simulink model "pmsm_sim"  (R2018a)
settings: Solver=ode15s  StartTime=0.0  StopTime=1  FixedStep=FastTsample / 10.  RelTol=1e-3
undefined symbols (not defined in the file): EncCntsToRads, MtrCtrlCal_T, MtrCtrlMd_T, MtrParams
libraries: powerlib x16, nesl_utility x12, fl_lib x10, pe_lib x5, pePwmGeneratorTwoLevel x1, powerlib_meascontrol x1
settings Model: Creator=elrobotista  LastModifiedBy=elrobotista
settings OptimizationCC: UseDivisionForNetSlopeComputation=on
settings ModelReferenceCC: EnableRefExpFcnMdlSchedulingChecks=off

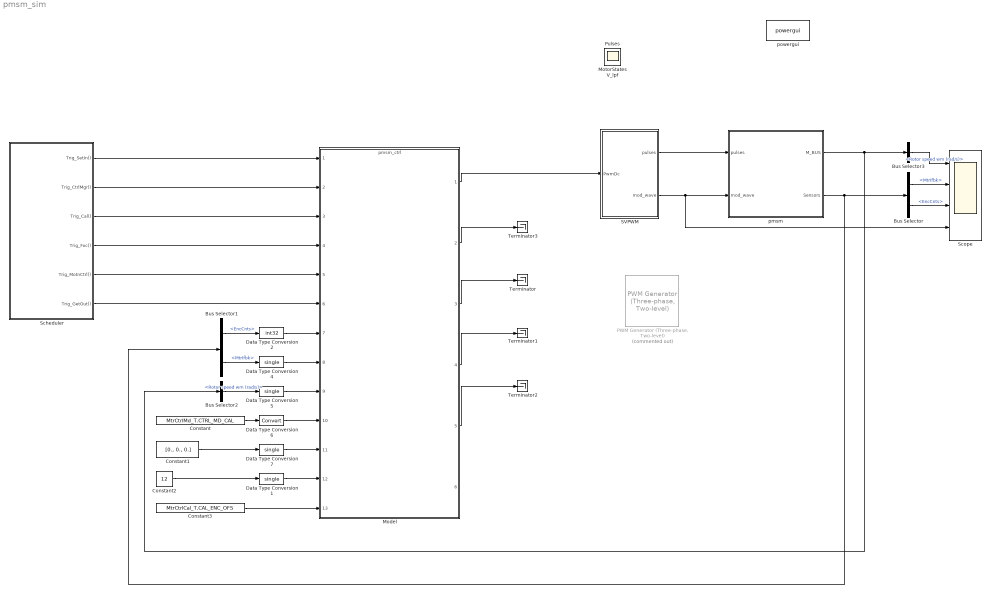
== system pmsm_sim ==
  " Scheduler" : Stateflow chart  TreatAsAtomicUnit=on  SystemSampleTime=1/30e3
  Bus Selector : BusSelector  OutputSignals=MtrIfbk,EncCnts
  Bus Selector1 : BusSelector  OutputSignals=EncCnts,MtrIfbk
  Bus Selector2 : BusSelector  OutputSignals=Rotor speed wm (rad/s)
  Bus Selector3 : BusSelector  OutputSignals=Rotor speed wm (rad/s)
  Constant : Constant  Value=MtrCtrlMd_T.CTRL_MD_CAL
  Constant1 : Constant  Value=[0., 0., 0.]
  Constant2 : Constant  Value=12
  Constant3 : Constant  Value=MtrCtrlCal_T.CAL_ENC_OFS
  Data Type Conversion{1,4..5,7} (4 alike) : DataTypeConversion  OutDataTypeStr=single
  Data Type Conversion2 : DataTypeConversion  OutDataTypeStr=int32
  Data Type Conversion6 : DataTypeConversion
  Model : ModelReference  ModelNameDialog=pmsm_ctrl  SimulationMode=Normal  ShowModelPeriodicEventPorts=on  ModelReferenceVersion=1.728
  "PWM Generator (Three-phase, Two-level)" : pePwmGeneratorTwoLevel/PWM Generator (Three-phase, Two-level)  Commented=on  OverrideUsingVariant=NaturalMode  PWMMode=Continuous PWM (CPWM)  CPWMMode=SPWM: sinusoidal PWM  DPWMMode=60 DPWM: 60 degree discontinuous PWM  fsw=30e3  Ts=5e-5
      settings: SamplingMode=Natural
  SVPWM : Subsystem
  Scope : Scope  NumInputPorts=4
  Terminator{,1..3} (4 alike) : Terminator
  pmsm : Subsystem  Variant=on  VariantControl=Variant1  OverrideUsingVariant=Variant1
  powergui : powerlib/powergui  Priority=1  SimulationMode=Continuous  SampleTime=50e-6  frequency=60  Iterations=50  frequencyindice=0  Pbase=100e6  ErrMax=1e-4  UnitsV=kV  UnitsW=MW  buscounter=0  FunctionMessages=off  echomessages=off  EnableUseOfTLC=off  CurrentSourceSwitches=off  DisableSnubberDevices=off  DisableRonSwitches=off  DisableVfSwitches=off  DisplayEquations=off  SolverType=Tustin/Backward Euler (TBE)  Interpol=off  ExternalGateDelay=off  methode=off  Ts=100  x0status=blocks  SPID=on  SwTol=0  HookPort=off  RestoreLinks=warning  ResistiveCurrentMeasurement=off  Frange=[0:2:500]  Ylog=off  Xlog=on  ShowGrid=off  save=off  variable=ZData  structure=0  ZoomFFT=off  StartTime=0.0  cycles=1  DisplayStyle=1  fundamental=60  FreqAxis=off  MaxFrequency=1000  frequencyindicesteady=1  RmsSteady=1  display=off
  MotorStates : Scope
  Pulses : Scope
  V_lpf : Scope
  wires:
  Bus Selector1/1 -> Data Type Conversion2/1  "<EncCnts>"
  Bus Selector1/2 -> Data Type Conversion4/1  "<MtrIfbk>"
  Constant/1 -> Data Type Conversion6/1
  Bus Selector2/1 -> Data Type Conversion5/1  "<Rotor speed wm (rad/s)>"
  Model/3 -> Terminator/1
  Model/4 -> Terminator1/1
  SVPWM/2(mod_wave) -> Scope/4, pmsm/2("mod_wave ")
  pmsm/1(" M_BUS") -> Bus Selector2/1, Bus Selector3/1
  pmsm/2(" Sensors") -> Bus Selector1/1, Bus Selector/1
  Constant1/1 -> Data Type Conversion7/1
  Model/5 -> Terminator2/1
  " Scheduler"/1(Trig_SetIn()) -> Model/1
  " Scheduler"/2(Trig_CtrlMgr()) -> Model/2
  " Scheduler"/3(Trig_Cal()) -> Model/3
  " Scheduler"/4(Trig_Foc()) -> Model/4
  " Scheduler"/5(Trig_MotnCtrl()) -> Model/5
  " Scheduler"/6(Trig_GetOut()) -> Model/6
  Data Type Conversion2/1 -> Model/7
  Data Type Conversion4/1 -> Model/8
  Data Type Conversion5/1 -> Model/9
  Data Type Conversion6/1 -> Model/10
  Data Type Conversion7/1 -> Model/11
  Data Type Conversion1/1 -> Model/12
  Model/1 -> SVPWM/1(PwmDc)
  Bus Selector/2 -> Scope/3  "<EncCnts>"
  Bus Selector/1 -> Scope/2  "<MtrIfbk>"
  Bus Selector3/1 -> Scope/1  "<Rotor speed wm (rad/s)>"
  Model/2 -> Terminator3/1
  SVPWM/1(pulses) -> pmsm/1("pulses ")
  Constant2/1 -> Data Type Conversion1/1
  Constant3/1 -> Model/13

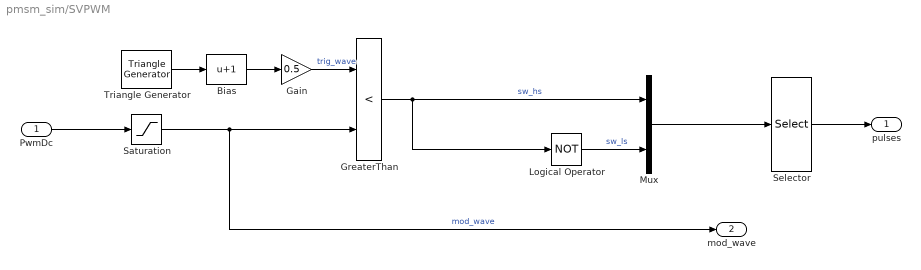
== system pmsm_sim/SVPWM ==
  PwmDc : Inport
  Bias : Bias  Bias=1
  Gain : Gain  Gain=0.5
  GreaterThan : RelationalOperator  Operator=<  OutDataTypeStr=boolean  RndMeth=Simplest
  Logical Operator : Logic  Operator=NOT  AllPortsSameDT=off  OutDataTypeStr=boolean
  Mux : Mux  Inputs=2
  Saturation : Saturate  UpperLimit=1  LowerLimit=0
  Selector : Selector  InputPortWidth=6  IndexOptions=Index vector (dialog)  Indices=[1 4 2 5 3 6]  OutputSizes=1
  Triangle Generator : powerlib_meascontrol/Pulse & Signal Generators/Triangle Generator  Freq=20e3  Phase=90  Ts=0
      settings: SourceProductName=Simscape Electrical
  pulses : Outport  VectorParamsAs1DForOutWhenUnconnected=on
  mod_wave : Outport  Port=2  VectorParamsAs1DForOutWhenUnconnected=on
  wires:
  Triangle Generator/1 -> Bias/1
  Bias/1 -> Gain/1
  Gain/1 -> GreaterThan/1  "trig_wave"
  Saturation/1 -> GreaterThan/2, mod_wave/1  "mod_wave"
  Logical Operator/1 -> Mux/2  "sw_ls"
  GreaterThan/1 -> Logical Operator/1, Mux/1  "sw_hs"
  PwmDc/1 -> Saturation/1
  Selector/1 -> pulses/1
  Mux/1 -> Selector/1

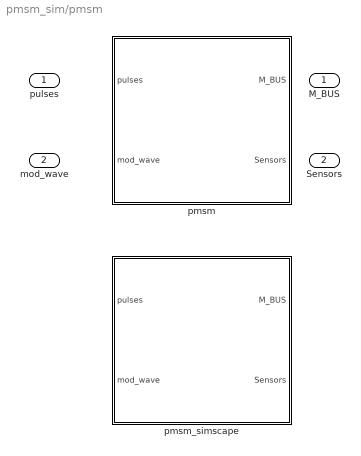
== system pmsm_sim/pmsm ==
  "pulses " : Inport
  "mod_wave " : Inport  Port=2
  pmsm : Subsystem  VariantControl=Variant2
  pmsm_simscape : Subsystem  VariantControl=Variant1
  " M_BUS" : Outport
  " Sensors" : Outport  Port=2

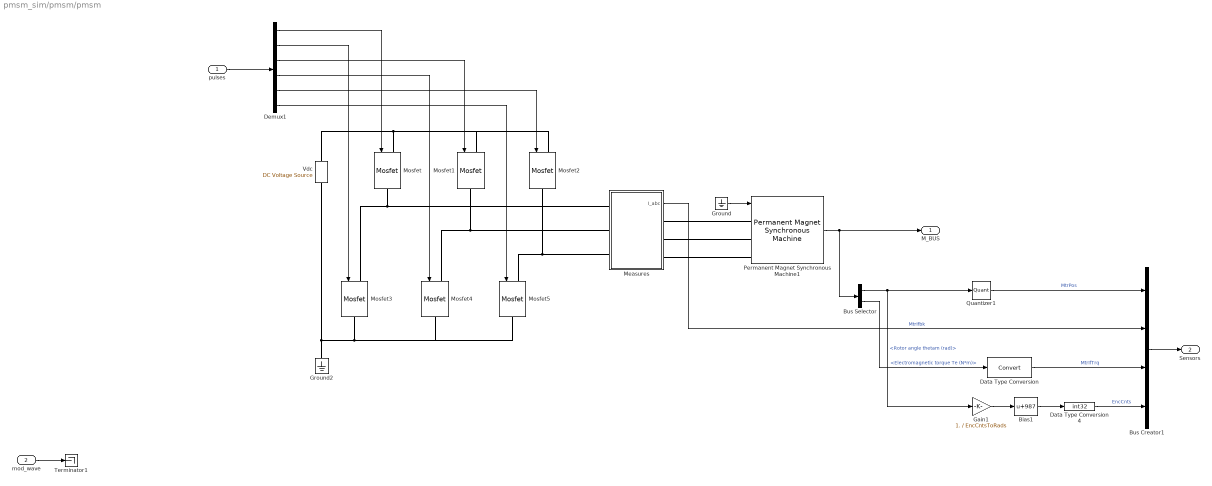
== system pmsm_sim/pmsm/pmsm ==
  pulses : Inport
  mod_wave : Inport  Port=2
  Bias1 : Bias  Bias=987
  Bus Creator1 : BusCreator  Inputs=4
  Bus Selector : BusSelector  OutputSignals=Rotor angle thetam (rad),Electromagnetic torque Te (N*m)
  Data Type Conversion : DataTypeConversion
  Data Type Conversion4 : DataTypeConversion  OutDataTypeStr=int32
  Demux1 : Demux  Outputs=6
  Gain1 : Gain  Gain=1. / EncCntsToRads  OutDataTypeStr=Inherit: Inherit via back propagation
      settings: AttributesFormatString=%<Gain>
  Ground : Ground
  Ground2 : powerlib/Elements/Ground  LConnTagsString=a
      settings: SourceProductName=Simscape Electrical
  Measures : Subsystem
  Mosfet{,1..5} (6 alike) : powerlib/Power Electronics/Mosfet  Ron=0.1  Lon=0  Rd=0.01  Vfd=0  IC=0  Rs=1e5  Cs=inf  Measurements=off
  Permanent Magnet Synchronous Machine1 : powerlib/Machines/Permanent Magnet Synchronous Machine  NbPhases=3  FluxDistribution=Sinusoidal  RotorType=Salient-pole  MechanicalLoad=Torque Tm  PresetModel=No  ShowDetailedParameters=on  MeasurementBus=off  Resistance=MtrParams.Rs  Inductance=8.5e-3  dqInductances=[MtrParams.Ld, MtrParams.Lq]  La=MtrParams.Ls  MachineConstant=Torque Constant (N.m / A_peak)  Flux=0.0058333  VoltageCst=4.2322  TorqueCst=MtrParams.Ktrq  Flat=120  Mechanical=[MtrParams.Jm, MtrParams.Kf, MtrParams.Poles, 0]  PolePairs=4  InitialConditions=[0,0, 0,0]  InitialConditions5ph=[0 0 0 0 0 0]  TsPowergui=0  TsBlock=-1  RefAngle=90 degrees behind phase A axis (modified Park)
  Quantizer1 : Quantizer  QuantizationInterval=2 * pi / MtrParams.EncCnts
  Terminator1 : Terminator
  Vdc : powerlib/Electrical Sources/DC Voltage Source  Amplitude=MtrParams.Vdc  Measurements=None
      settings: SourceProductName=Simscape Electrical
  M_BUS : Outport
  Sensors : Outport  Port=2
  wires:
  Ground/1 -> Permanent Magnet Synchronous Machine1/1
  Permanent Magnet Synchronous Machine1/1 -> Bus Selector/1, M_BUS/1
  Bus Selector/1 -> Quantizer1/1, Gain1/1  "<Rotor angle thetam (rad)>"
  Measures/1(I_abc) -> Bus Creator1/2  "MtrIfbk"
  pulses/1 -> Demux1/1
  Quantizer1/1 -> Bus Creator1/1  "MtrPos"
  Bias1/1 -> Data Type Conversion4/1
  Gain1/1 -> Bias1/1
  Bus Selector/2 -> Data Type Conversion/1  "<Electromagnetic torque Te (N*m)>"
  Bus Creator1/1 -> Sensors/1
  Data Type Conversion4/1 -> Bus Creator1/4  "EncCnts"
  Data Type Conversion/1 -> Bus Creator1/3  "MtrIfTrq"
  mod_wave/1 -> Terminator1/1
  Demux1/1 -> Mosfet/1
  Demux1/2 -> Mosfet3/1
  Demux1/3 -> Mosfet1/1
  Demux1/4 -> Mosfet4/1
  Demux1/5 -> Mosfet2/1
  Demux1/6 -> Mosfet5/1
  connections:
  Permanent Magnet Synchronous Machine1/LConn3 -- Measures/RConn3
  Permanent Magnet Synchronous Machine1/LConn2 -- Measures/RConn2
  Permanent Magnet Synchronous Machine1/LConn1 -- Measures/RConn1
  Mosfet5/RConn1 -- Mosfet4/RConn1 -- Mosfet3/RConn1 -- Vdc/LConn1 -- Ground2/LConn1
  Mosfet5/LConn1 -- Measures/LConn3 -- Mosfet2/RConn1
  Mosfet2/LConn1 -- Mosfet1/LConn1 -- Mosfet/LConn1 -- Vdc/RConn1
  Mosfet4/LConn1 -- Measures/LConn2 -- Mosfet1/RConn1
  Mosfet3/LConn1 -- Measures/LConn1 -- Mosfet/RConn1

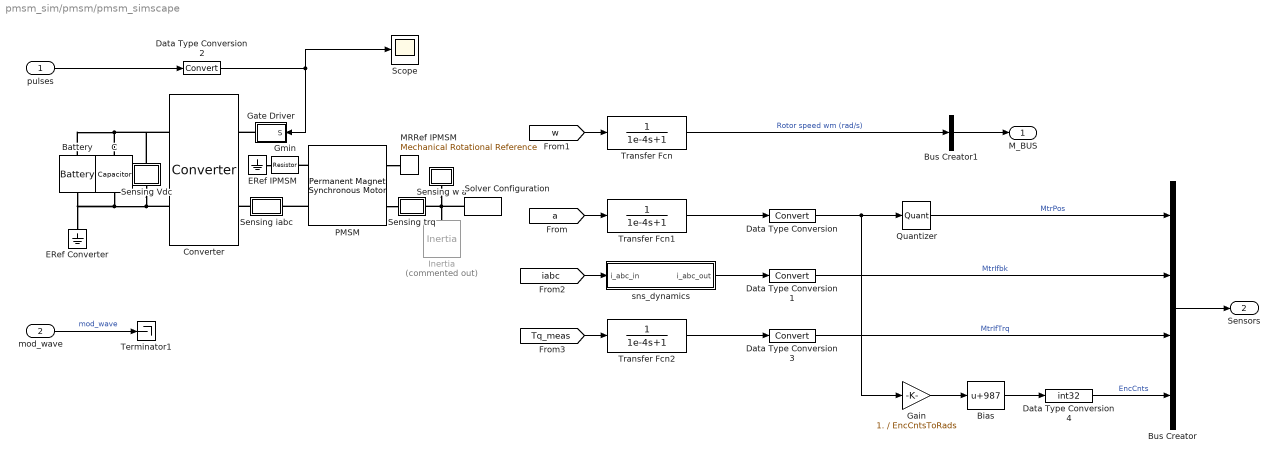
== system pmsm_sim/pmsm/pmsm_simscape ==
  pulses : Inport
  mod_wave : Inport  Port=2
  Battery : pe_lib/Sources/Battery  Vnom=MtrParams.Vdc V  R1=0.001 Ohm  prm_AH=1  AH=200 hr*A  V1=290 V  AH1=50 hr*A  prm_R2=1  R2=2000 Ohm  prm_dyn=1  Rp1=0.005 Ohm  tau1=30 s  Rp2=0.005 Ohm  tau2=30 s  prm_fade=1  N_fade=100  AH_fade=45 hr*A  R1_fade=2.02 Ohm  V1_fade=10.35 V  i_specify=off  i_priority=None  i=0 A  i_nominal_specify=off  i_nominal_unit=A  i_nominal_value=1  v_specify=off  v_priority=None  v=0 V  v_nominal_specify=off  v_nominal_unit=V  v_nominal_value=1  charge_specify=on  charge_priority=High  charge=200 hr*A  charge_nominal_specify=off  charge_nominal_unit=hr*A  charge_nominal_value=1  num_cycles_specify=off  num_cycles_priority=High  num_cycles=0  num_cycles_nominal_specify=off  num_cycles_nominal_unit=1  num_cycles_nominal_value=1  thermal_mass=30000 J/K  Tmeas=298.15 K  Vnom_T2=12 V  R1_T2=2.2 Ohm  V1_T2=11.4 V  R2_T2=2200 Ohm  Rp1_T2=0.005 Ohm  tau1_T2=30 s  Rp2_T2=0.005 Ohm  tau2_T2=30 s  Tmeas2=273.15 K  temperature_specify=off  temperature_priority=High  temperature=298.15 K  temperature_nominal_specify=off  temperature_nominal_unit=K  temperature_nominal_value=1
      settings: SourceProductName=Simscape Power Systems  SourceProductBaseCode=PS
  Bias : Bias  Bias=987
  Bus Creator : BusCreator  Inputs=4
  Bus Creator1 : BusCreator  Inputs=1
  C : fl_lib/Electrical/Electrical Elements/Capacitor  c=1e-3 F  r=1e-6 Ohm  g=0 1/Ohm  i_specify=off  i_priority=None  i=0 A  i_nominal_specify=off  i_nominal_unit=A  i_nominal_value=1  v_specify=off  v_priority=None  v=0 V  v_nominal_specify=off  v_nominal_unit=V  v_nominal_value=1  vc_specify=off  vc_priority=High  vc=0 V  vc_nominal_specify=off  vc_nominal_unit=V  vc_nominal_value=1
      settings: SourceProductName=Foundation Library
  Converter : pe_lib/Semiconductors/Converter  device_type=2  Vf=0.8 V  Ron=0.001 Ohm  Rds=0.001 Ohm  Goff=1e-5 1/Ohm  Vth=0.01 V  Vgt=1 V  Vgt_off=-1 V  Ih=1 A  diode_param=2  diode_Vf=0.8 V  diode_Ron=0.001 Ohm  diode_Goff=1e-5 1/Ohm  diode_C=50 nF  diode_iRM=-235 A  diode_iF=300 A  diode_idot=-50 A/us  diode_trr_param=1  diode_trr_factor=3  diode_trr=15 us  diode_Qrr=1.5e+3 s*uA  snubber_type=0  Rs=0.1 Ohm  Cs=1e-7 F
      settings: SourceProductName=Simscape Power Systems  SourceProductBaseCode=PS
  Data Type Conversion{,1..3} (4 alike) : DataTypeConversion
  Data Type Conversion4 : DataTypeConversion  OutDataTypeStr=int32
  ERef Converter : fl_lib/Electrical/Electrical Elements/Electrical Reference
      settings: SourceProductName=Foundation Library
  ERef IPMSM : fl_lib/Electrical/Electrical Elements/Electrical Reference
      settings: SourceProductName=Foundation Library
  Gain : Gain  Gain=1. / EncCntsToRads  OutDataTypeStr=Inherit: Inherit via back propagation
      settings: AttributesFormatString=%<Gain>
  Gate Driver : Subsystem
  Gmin : fl_lib/Electrical/Electrical Elements/Resistor  R=1e9 Ohm  i_specify=off  i_priority=High  i=0 A  i_nominal_specify=off  i_nominal_unit=A  i_nominal_value=1  v_specify=off  v_priority=High  v=0 V  v_nominal_specify=off  v_nominal_unit=V  v_nominal_value=1
      settings: SourceProductName=Foundation Library
  Inertia : fl_lib/Mechanical/Rotational Elements/Inertia  Commented=on  inertia=MtrParams.Jm kg*m^2  w_specify=on  w_priority=High  w=0 rpm  w_nominal_specify=off  w_nominal_unit=rad/s  w_nominal_value=1  t_specify=off  t_priority=High  t=0 N*m  t_nominal_specify=off  t_nominal_unit=N*m  t_nominal_value=1
      settings: SourceProductName=Foundation Library
  MRRef IPMSM : fl_lib/Mechanical/Rotational Elements/Mechanical Rotational Reference
      settings: SourceProductName=Foundation Library
  PMSM : pe_lib/Machines/Permanent Magnet Rotor/Permanent Magnet Synchronous Motor  nPolePairs=MtrParams.Poles  pmflux_param=2  pm_flux_linkage=MtrParams.MFlux Wb  torque_constant=MtrParams.Ktrq N*m/A  back_emf_constant=0.18 V/(rad/s)  stator_param=1  Ld=MtrParams.Ld H  Lq=MtrParams.Lq H  L0=0 H  Ls=0.0002 H  Lm=0.00002 H  Ms=0.00002 H  Rs=MtrParams.Rs Ohm  zero_sequence=pe.enum.park.zerosequence.include  J=MtrParams.Jm kg*m^2  lam=0 N*m/(rad/s)  axes_param=1  i_d_specify=off  i_d_priority=None  i_d=0 A  i_d_nominal_specify=off  i_d_nominal_unit=A  i_d_nominal_value=1  i_q_specify=off  i_q_priority=None  i_q=0 A  i_q_nominal_specify=off  i_q_nominal_unit=A  i_q_nominal_value=1  torque_specify=off  torque_priority=None  torque=0 N*m  torque_nominal_specify=off  torque_nominal_unit=N*m  torque_nominal_value=1  angular_velocity_specify=on  angular_velocity_priority=None  angular_velocity=0 rpm  angular_velocity_nominal_specify=off  angular_velocity_nominal_unit=rpm  angular_velocity_nominal_value=1  angular_position_specify=on  angular_position_priority=High  angular_position=0 rad  angular_position_nominal_specify=off  angular_position_nominal_unit=deg  angular_position_nominal_value=1
      settings: SourceProductName=Simscape Power Systems  SourceProductBaseCode=PS
  Quantizer : Quantizer  QuantizationInterval=2 * pi / MtrParams.EncCnts
  Scope : Scope
  Sensing Vdc : Subsystem
      mask Display: disp('vdc')
  Sensing trq : Subsystem
      mask Display: disp('trq')
  Sensing w a : Subsystem
      mask Display: disp('w,a')
  Sensing iabc : Subsystem
      mask Display: disp('iabc')
  Solver Configuration : nesl_utility/Solver Configuration  PhysicalDomain=network_engine_domain  SubClassName=solver  LeftPortType=input  RightPortType=generic  Tones=[]  Harmonics=[]  SimulateNoise=off  Profile=off  UseLocalSampling=off  EnableSwitchedLinearOptims=on  FrequencyDomain=off  UseCCode=off  RelTol=0.001  AbsTol=1e-06  MinStep=1e-09  ToWorkspace=off  RevertToSquareIcSolve=off  NumHomotopyIterations=100  PhasorMode=off  PhasorModeNumHarmonics=1  DoDC=off  ResidualTolerance=1e-9  UseLocalSolver=on  LocalSolverChoice=NE_BACKWARD_EULER_ADVANCER  LocalSolverSampleTime=SimParams.Ts  DoFixedCost=on  MaxNonlinIter=4  MaxModeIter=2  LinearAlgebra=Sparse  EquationFormulation=NE_TIME_EF  DelaysMemoryBudget=1024  AutomaticFiltering=on  FilteringTimeConstant=0.001
  Terminator1 : Terminator
  Transfer Fcn : TransferFcn  Denominator=[1e-4 1]
  Transfer Fcn1 : TransferFcn  Denominator=[1e-4 1]
  Transfer Fcn2 : TransferFcn  Denominator=[1e-4 1]
  sns_dynamics : Subsystem
  M_BUS : Outport
  Sensors : Outport  Port=2
  wires:
  Bus Creator/1 -> Sensors/1
  mod_wave/1 -> Terminator1/1  "mod_wave"
  [a] -> Transfer Fcn1/1
  Data Type Conversion1/1 -> Bus Creator/2  "MtrIfbk"
  Bus Creator1/1 -> M_BUS/1
  [w] -> Transfer Fcn/1
  Data Type Conversion2/1 -> Scope/1, Gate Driver/1(S)
  pulses/1 -> Data Type Conversion2/1
  Transfer Fcn/1 -> Bus Creator1/1  "Rotor speed wm (rad/s)"
  [iabc] -> sns_dynamics/1(i_abc_in)
  sns_dynamics/1(i_abc_out) -> Data Type Conversion1/1
  [Tq_meas] -> Transfer Fcn2/1
  Transfer Fcn2/1 -> Data Type Conversion3/1
  Data Type Conversion3/1 -> Bus Creator/3  "MtrIfTrq"
  Data Type Conversion/1 -> Gain/1, Quantizer/1
  Gain/1 -> Bias/1
  Transfer Fcn1/1 -> Data Type Conversion/1
  Data Type Conversion4/1 -> Bus Creator/4  "EncCnts"
  Quantizer/1 -> Bus Creator/1  "MtrPos"
  Bias/1 -> Data Type Conversion4/1
  connections:
  Sensing w a/LConn1 -- Sensing trq/RConn1 -- Solver Configuration/RConn1 -- Inertia/LConn1
  C/LConn1 -- Battery/LConn1 -- Converter/RConn1 -- Sensing Vdc/LConn1
  Sensing Vdc/RConn1 -- Battery/RConn1 -- ERef Converter/LConn1 -- C/RConn1 -- Converter/RConn2
  PMSM/LConn1 -- Sensing iabc/RConn1
  ERef IPMSM/LConn1 -- Gmin/LConn1
  PMSM/RConn1 -- Sensing trq/LConn1
  Gate Driver/RConn1 -- Converter/LConn1
  Sensing iabc/LConn1 -- Converter/LConn2
  PMSM/RConn2 -- MRRef IPMSM/LConn1
  PMSM/LConn2 -- Gmin/RConn1

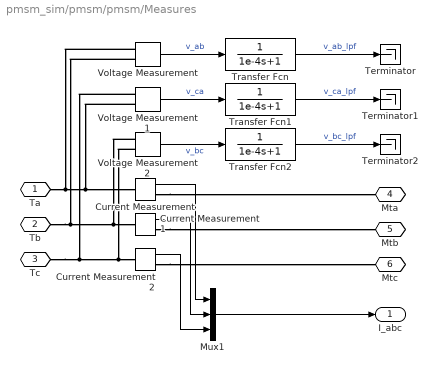
== system pmsm_sim/pmsm/pmsm/Measures ==
  Current Measurement : powerlib/Measurements/Current Measurement  Tag=PoWeRsYsTeMmEaSuReMeNt  PhasorSimulation=off  OutputType=Magnitude  PSBequivalent=0
      settings: SourceProductName=Simscape Electrical
  Current Measurement1 : powerlib/Measurements/Current Measurement  Tag=PoWeRsYsTeMmEaSuReMeNt  PhasorSimulation=off  OutputType=Magnitude  PSBequivalent=0
      settings: SourceProductName=Simscape Electrical
  Current Measurement2 : powerlib/Measurements/Current Measurement  Tag=PoWeRsYsTeMmEaSuReMeNt  PhasorSimulation=off  OutputType=Magnitude  PSBequivalent=0
      settings: SourceProductName=Simscape Electrical
  Mux1 : Mux  Inputs=3
  Terminator : Terminator
  Terminator1 : Terminator
  Terminator2 : Terminator
  Transfer Fcn : TransferFcn  Denominator=[1e-4 1]
  Transfer Fcn1 : TransferFcn  Denominator=[1e-4 1]
  Transfer Fcn2 : TransferFcn  Denominator=[1e-4 1]
  Voltage Measurement : powerlib/Measurements/Voltage Measurement  PhasorSimulation=off  OutputType=Complex  PSBequivalent=0
      settings: SourceProductName=Simscape Electrical
  Voltage Measurement1 : powerlib/Measurements/Voltage Measurement  PhasorSimulation=off  OutputType=Complex  PSBequivalent=0
      settings: SourceProductName=Simscape Electrical
  Voltage Measurement2 : powerlib/Measurements/Voltage Measurement  PhasorSimulation=off  OutputType=Complex  PSBequivalent=0
      settings: SourceProductName=Simscape Electrical
  Ta : PMIOPort  Side=Left
  Tb : PMIOPort  Port=2  Side=Left
  Tc : PMIOPort  Port=3  Side=Left
  Mta : PMIOPort  Port=4  Side=Right
  Mtb : PMIOPort  Port=5  Side=Right
  Mtc : PMIOPort  Port=6  Side=Right
  I_abc : Outport
  wires:
  Current Measurement1/1 -> Mux1/2
  Current Measurement/1 -> Mux1/1
  Current Measurement2/1 -> Mux1/3
  Mux1/1 -> I_abc/1
  Voltage Measurement/1 -> Transfer Fcn/1  "v_ab"
  Voltage Measurement1/1 -> Transfer Fcn1/1  "v_ca"
  Voltage Measurement2/1 -> Transfer Fcn2/1  "v_bc"
  Transfer Fcn/1 -> Terminator/1  "v_ab_lpf"
  Transfer Fcn1/1 -> Terminator1/1  "v_ca_lpf"
  Transfer Fcn2/1 -> Terminator2/1  "v_bc_lpf"
  connections:
  Current Measurement1/RConn1 -- Mtb/RConn1
  Tb/RConn1 -- Voltage Measurement2/LConn1 -- Current Measurement1/LConn1 -- Voltage Measurement/LConn2
  Current Measurement/RConn1 -- Mta/RConn1
  Ta/RConn1 -- Current Measurement/LConn1 -- Voltage Measurement1/LConn2 -- Voltage Measurement/LConn1
  Tc/RConn1 -- Voltage Measurement2/LConn2 -- Current Measurement2/LConn1 -- Voltage Measurement1/LConn1
  Current Measurement2/RConn1 -- Mtc/RConn1

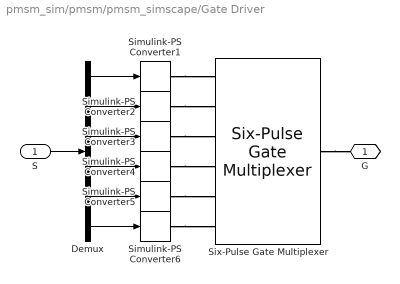
== system pmsm_sim/pmsm/pmsm_simscape/Gate Driver ==
  S : Inport
  Demux : Demux  Outputs=6
  Simulink-PS Converter{1..6} (6 alike) : nesl_utility/Simulink-PS Converter  PhysicalDomain=network_engine_domain  SubClassName=ps_input  LeftPortType=input  RightPortType=output  PseudoPeriodic=off  Frequencies=[]  NoiseDistribution=none  NoiseParameters=[]  Unit=1  AffineConversion=off  FilteringAndDerivatives=zero  SimscapeFilterOrder=1  InputFilterTimeConstant=0.001  UdotUserProvided=1
  Six-Pulse Gate Multiplexer : pe_lib/Semiconductors/Six-Pulse Gate Multiplexer  R=0 Ohm
      settings: SourceProductName=Simscape Power Systems  SourceProductBaseCode=PS
  G : PMIOPort  Side=Right
  wires:
  Demux/1 -> Simulink-PS Converter1/1
  S/1 -> Demux/1
  Demux/4 -> Simulink-PS Converter4/1
  Demux/2 -> Simulink-PS Converter2/1
  Demux/3 -> Simulink-PS Converter3/1
  Demux/5 -> Simulink-PS Converter5/1
  Demux/6 -> Simulink-PS Converter6/1
  connections:
  Six-Pulse Gate Multiplexer/RConn1 -- G/RConn1
  Simulink-PS Converter1/RConn1 -- Six-Pulse Gate Multiplexer/LConn1
  Simulink-PS Converter3/RConn1 -- Six-Pulse Gate Multiplexer/LConn3
  Simulink-PS Converter5/RConn1 -- Six-Pulse Gate Multiplexer/LConn5
  Simulink-PS Converter6/RConn1 -- Six-Pulse Gate Multiplexer/LConn6
  Simulink-PS Converter4/RConn1 -- Six-Pulse Gate Multiplexer/LConn4
  Simulink-PS Converter2/RConn1 -- Six-Pulse Gate Multiplexer/LConn2

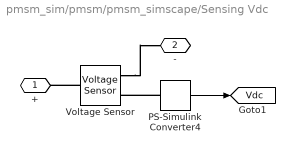
== system pmsm_sim/pmsm/pmsm_simscape/Sensing Vdc ==
  PS-Simulink Converter4 : nesl_utility/PS-Simulink Converter  PhysicalDomain=network_engine_domain  SubClassName=ps_output  LeftPortType=input  RightPortType=output  PseudoPeriodic=off  Frequencies=[]  Unit=V  AffineConversion=off
  Voltage Sensor : fl_lib/Electrical/Electrical Sensors/Voltage Sensor
      settings: SourceProductName=Foundation Library
  + : PMIOPort  Side=Left
  - : PMIOPort  Port=2  Side=Right
  tag scope: Vdc=global
  wires:
  PS-Simulink Converter4/1 -> [Vdc]
  connections:
  Voltage Sensor/LConn1 -- +/RConn1
  Voltage Sensor/RConn2 -- -/RConn1
  PS-Simulink Converter4/LConn1 -- Voltage Sensor/RConn1

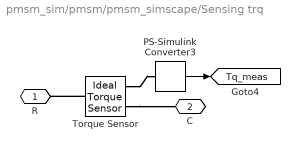
== system pmsm_sim/pmsm/pmsm_simscape/Sensing trq ==
  PS-Simulink Converter3 : nesl_utility/PS-Simulink Converter  PhysicalDomain=network_engine_domain  SubClassName=ps_output  LeftPortType=input  RightPortType=output  PseudoPeriodic=off  Frequencies=[]  Unit=N*m  AffineConversion=off
  Torque Sensor : fl_lib/Mechanical/Mechanical Sensors/Ideal Torque Sensor
      settings: SourceProductName=Foundation Library
  R : PMIOPort  Side=Left
  C : PMIOPort  Port=2  Side=Right
  tag scope: Tq_meas=global
  wires:
  PS-Simulink Converter3/1 -> [Tq_meas]
  connections:
  Torque Sensor/RConn1 -- C/RConn1
  Torque Sensor/RConn2 -- PS-Simulink Converter3/LConn1
  Torque Sensor/LConn1 -- R/RConn1

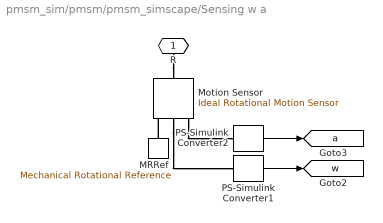
== system pmsm_sim/pmsm/pmsm_simscape/Sensing w a ==
  MRRef : fl_lib/Mechanical/Rotational Elements/Mechanical Rotational Reference
      settings: SourceProductName=Foundation Library
  Motion Sensor : fl_lib/Mechanical/Mechanical Sensors/Ideal Rotational Motion Sensor  offset=0 deg
      settings: SourceProductName=Foundation Library
  PS-Simulink Converter1 : nesl_utility/PS-Simulink Converter  PhysicalDomain=network_engine_domain  SubClassName=ps_output  LeftPortType=input  RightPortType=output  PseudoPeriodic=off  Frequencies=[]  Unit=rad/s  AffineConversion=off
  PS-Simulink Converter2 : nesl_utility/PS-Simulink Converter  PhysicalDomain=network_engine_domain  SubClassName=ps_output  LeftPortType=input  RightPortType=output  PseudoPeriodic=off  Frequencies=[]  Unit=rad  AffineConversion=off
  R : PMIOPort  Side=Left
  tag scope: a=global, w=global
  wires:
  PS-Simulink Converter1/1 -> [w]
  PS-Simulink Converter2/1 -> [a]
  connections:
  R/RConn1 -- Motion Sensor/LConn1
  Motion Sensor/RConn2 -- PS-Simulink Converter1/LConn1
  MRRef/LConn1 -- Motion Sensor/RConn1
  Motion Sensor/RConn3 -- PS-Simulink Converter2/LConn1

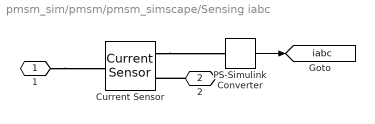
== system pmsm_sim/pmsm/pmsm_simscape/Sensing iabc ==
  Current Sensor : pe_lib/Sensors/Current Sensor
      settings: SourceProductName=Simscape Power Systems  SourceProductBaseCode=PS
  PS-Simulink Converter : nesl_utility/PS-Simulink Converter  PhysicalDomain=network_engine_domain  SubClassName=ps_output  LeftPortType=input  RightPortType=output  PseudoPeriodic=off  Frequencies=[]  Unit=A  AffineConversion=off
  1 : PMIOPort  Side=Left
  2 : PMIOPort  Port=2  Side=Right
  tag scope: iabc=global
  wires:
  PS-Simulink Converter/1 -> [iabc]
  connections:
  1/RConn1 -- Current Sensor/LConn1
  2/RConn1 -- Current Sensor/RConn2
  Current Sensor/RConn1 -- PS-Simulink Converter/LConn1

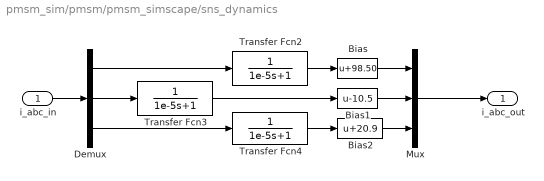
== system pmsm_sim/pmsm/pmsm_simscape/sns_dynamics ==
  i_abc_in : Inport
  Bias : Bias  Bias=98.50
  Bias1 : Bias  Bias=-10.5
  Bias2 : Bias  Bias=20.9
  Demux : Demux  Outputs=3
  Mux : Mux  Inputs=3
  Transfer Fcn2 : TransferFcn  Denominator=[1e-5 1]
  Transfer Fcn3 : TransferFcn  Denominator=[1e-5 1]
  Transfer Fcn4 : TransferFcn  Denominator=[1e-5 1]
  i_abc_out : Outport
  wires:
  Demux/1 -> Transfer Fcn2/1
  Demux/2 -> Transfer Fcn3/1
  Transfer Fcn3/1 -> Bias1/1
  Demux/3 -> Transfer Fcn4/1
  Transfer Fcn4/1 -> Bias2/1
  Mux/1 -> i_abc_out/1
  Transfer Fcn2/1 -> Bias/1
  i_abc_in/1 -> Demux/1
  Bias/1 -> Mux/1
  Bias1/1 -> Mux/2
  Bias2/1 -> Mux/3

== stateflow chart pmsm_sim/ Scheduler ==
  (default) -> (junction 26)
  (junction 26) -> (junction 25) [order 1] : [cnt == 0]
  (junction 25) -> (junction 1)
  (junction 26) -> (junction 1) [order 2]
  (junction 1) -> (junction 15) [order 1] : [!(cnt %% TASK_COUNT_30KHZ)]{Trig_SetIn; Trig_Foc; Trig_GetOut;}
  (junction 15) -> (junction 9)
  (junction 1) -> (junction 9) [order 2]
  (junction 9) -> (junction 18) [order 1] : [!(cnt %% TASK_COUNT_1KHZ)] {Trig_CtrlMgr; Trig_Cal; Trig_MotnCtrl;}
  (junction 18) -> (junction 19) : {cnt = 1;}
  (junction 9) -> (junction 19) [order 2] : {cnt++;}
  data: TASK_COUNT_1KHZ constant uint32 size=1 =30; TASK_COUNT_30KHZ constant uint32 size=1 =1; cnt local uint32 size=1 =0; dbg_out local double
  events: Trig_SetIn output FUNCTION_CALL_EVENT; Trig_CtrlMgr output FUNCTION_CALL_EVENT; Trig_Cal output FUNCTION_CALL_EVENT; Trig_Foc output FUNCTION_CALL_EVENT; Trig_MotnCtrl output FUNCTION_CALL_EVENT; Trig_GetOut output FUNCTION_CALL_EVENT
